simulink model "genericStructBusObject"  (Simulink 6.6)
settings: Solver=FixedStepDiscrete  StartTime=0.0  StopTime=10.0  FixedStep=1  RelTol=1e-3
PreLoadFcn:
  | myGSBO
settings Model: Creator=hnine  LastModifiedBy=hnine

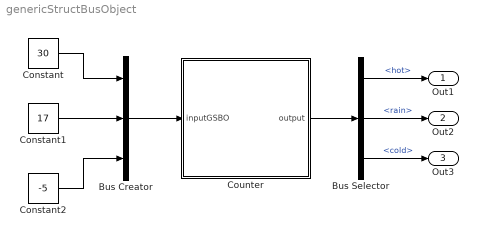
== system genericStructBusObject ==
  Bus Creator : BusCreator  Inputs=3
  Bus Selector : BusSelector  OutputSignals=hot,rain,cold
  Constant : Constant  Value=30  OutDataTypeMode=double
  Constant1 : Constant  Value=17  OutDataTypeMode=double
  Constant2 : Constant  Value=-5  OutDataTypeMode=double
  Counter : Stateflow chart
  Out1 : Outport
  Out2 : Outport  Port=2
  Out3 : Outport  Port=3
  wires:
  Constant/1 -> Bus Creator/1
  Constant1/1 -> Bus Creator/2
  Constant2/1 -> Bus Creator/3
  Bus Creator/1 -> Counter/1(inputGSBO)
  Counter/1(output) -> Bus Selector/1
  Bus Selector/1 -> Out1/1  "<hot>"
  Bus Selector/2 -> Out2/1  "<rain>"
  Bus Selector/3 -> Out3/1  "<cold>"

== stateflow chart Counter ==
  state s1
  (default) -> s1
  s1 -> s1 [order 1] : [ ctr < 4] / ctr = ctr+1;
      | output.rain = inputGSBO.rain + ctr;
      | output.hot = inputGSBO.hot - ctr;
      | output.cold = inputGSBO.cold * ctr;
  s1 -> s1 [order 2] : [ctr >= 4] / ctr = 0;
      | output.rain = 25;
      | output.hot = 50;
      | output.cold = -25
  data: inputGSBO input gsbo =0; output output gsbo; ctr local uint32
